simulink model "TV2016"  (Simulink 8.5)
settings: Solver=FixedStepDiscrete  StartTime=0.0  StopTime=inf  FixedStep=0.001  RelTol=1e-3
PreLoadFcn:
  | FSE_Parameters
values from neighbouring files (symbols this model uses):
  car_params = Simulink_Car_params    [TV2016_parameters.m]
  i_Diff = 15.47    [TV2016_parameters.m]
  Kp = 1    [TV2016_parameters.m]
  powerLimitControl = Simulink_el    [TV2016_parameters.m]
  settings = Simulink_Settings    [TV2016_parameters.m]
  SpdC_BCC = 0    [TV2016_parameters.m]
  Speed_Neg_sat = -21    [TV2016_parameters.m]
  Speed_Pos_sat = 21    [TV2016_parameters.m]
  speedEstimation = Simulink_speedEst    [TV2016_parameters.m]
  Tn_n = 0    [TV2016_parameters.m]
  tractionControl = Simulink_tc    [TV2016_parameters.m]
  Use_Joystick = 1    [TV2016_parameters.m]
  yawRateControl = Simulink_yawRate    [TV2016_parameters.m]
libraries: CarMaker4SL x174, simulink x27, simulink_extras x14
(part 5 of 5)

== matlab function CarMaker/Estimations/EstimateVx/velocity_Estimation ==
  data: sensors input Bus: SensorInputs; V_est_x output double; normalForces input Bus: normalForces; settings parameter double; car_params parameter double; speedEstimation parameter double
function V_est_x  = velocityEstimation(sensors,normalForces,settings,car_params,speedEstimation)
%#codegen


persistent firstIteration;
persistent v;
persistent error;
persistent K;
persistent drift;

k_FL = single(0); % Gain 
k_FR = single(0); % Gain
k_RL = single(0); % Gain
k_RR = single(0); % Gain
% Gains for trusting, not trusting wheel speed measurements
Hg = speedEstimation.High_gain;
Lg = speedEstimation.Low_gain;
% Variances
all_Var = single(0); % Variance for all measurements
front_rear_Var = single(0);
front_Var = single(0);
rear_Var = single(0);
left_Var = single(0);
right_Var = single(0);
% LIMITS:
velocity_deviation_limit = speedEstimation.velocity_deviation_limit;
lim = speedEstimation.variance_limit;
RPM_derivative_limit = speedEstimation.RPM_derivative_limit;

% Measurement vector
C = [1;1;1;1]; % Create four copies of predicted vx


c = single(2*pi/(car_params.GR*60));

t = settings.control_system_sample_time;
%Weights taken from wikipedia
%sg_Weight = single( [ 1; -8; 0; 8; -1] );
sg_Weight = single( [ -1; 8; 0; -8; 1] );
%sg_Weight = single([0.3; 0.1; -0.1 ; -0.3]);
%sg_Weight = single([1; -1; 0 ; -0]);
% ------------------------------
% COPY VARIABLES EACH TIMESTEP
% ------------------------------
S = sensors.steering_wheel_angle; % Steering angle in rad( Mean of front wheels)
ax = sensors.ax; % Should be true linear acceleration compensated for roll angle
%Fz, used to determine what wheel speeds to trust.
Fz = [normalForces.FL, normalForces.FR, normalForces.RL ,normalForces.RR];
% Determine CoG Vx from motor RPM. Simple atm. Not considering vy.
Whl_v_FL = sensors.RPM_FL*c*car_params.r_eff*cos(S) + sensors.yawRate*car_params.t_f;
Whl_v_FR = sensors.RPM_FR*c*car_params.r_eff*cos(S) - sensors.yawRate*car_params.t_f;
Whl_v_RL = sensors.RPM_RL*c*car_params.r_eff + sensors.yawRate*car_params.t_r;
Whl_v_RR = sensors.RPM_RR*c*car_params.r_eff - sensors.yawRate*car_params.t_r;
whl_speed.v_FL = Whl_v_FL;
whl_speed.v_FR = Whl_v_FR;
whl_speed.v_RL = Whl_v_RL;
whl_speed.v_RR = Whl_v_RR;


RPM = [sensors.RPM_FL, sensors.RPM_FR, sensors.RPM_RL, sensors.RPM_RR]';
% Measurement vector, compensated RPMS
Y_meas = [Whl_v_FL, Whl_v_FR, Whl_v_RL, Whl_v_RR]';
% Input Derivative of RPM
rateRPM_FL = sensors.RPM_der_FL;
rateRPM_FR = sensors.RPM_der_FR;
rateRPM_RL = sensors.RPM_der_RL;
rateRPM_RR = sensors.RPM_der_RR;

% Different sums of normal forces, used to determine what wheels to trust
left_Fz = sum(Fz([1 3]));
right_Fz = sum(Fz([2 4]));
front_Fz = sum(Fz(1:2));
rear_Fz = sum(Fz(3:4));
% ALGORITHM
if (isempty(firstIteration))
    K = single(ones(1,4));
    v = single(0);
    V_est_x = v;
    error = Y_meas- C*v;
    firstIteration = 2;
    drift = single(0);
else
    v_ins = sensors.V_x_INS + 0.05 + drift;
    mean_WhlV = max(0.001,mean(Y_meas));
    mean_front_WhlV = max(0.001,mean(Y_meas(1:2)));
    mean_rear_WhlV  = max(0.001,mean(Y_meas(3:4)));
    mean_left_WhlV  = max(0.001,mean(Y_meas([1 3])));
    mean_right_WhlV = max(0.001,mean(Y_meas([2 4])));

    all_Var = var(Y_meas,1)/mean_WhlV;
    front_rear_Var = var([mean_front_WhlV, mean_rear_WhlV],1)/mean_WhlV;
    front_Var = var(Y_meas(1:2),1)/mean_front_WhlV;
    rear_Var  = var(Y_meas(3:4),1)/mean_rear_WhlV;
    
    left_Var    = var(Y_meas([1 3]),1)/mean_left_WhlV;
    right_Var   = var(Y_meas([2 4]),1)/mean_right_WhlV;   
    
    if ( (abs(Whl_v_FL - v_ins) > velocity_deviation_limit)...
       && (abs(Whl_v_FR - v_ins) > velocity_deviation_limit)...
       && (abs(Whl_v_RL - v_ins) > velocity_deviation_limit)...
       && (abs(Whl_v_RR - v_ins) > velocity_deviation_limit) )
        
        K = [Lg, Lg, Lg, Lg];
    elseif (all_Var  < lim ) 
        % low variance for all wheels.
        % Check derivative of motor RPM
        if ( (rateRPM_FL > RPM_derivative_limit) ||...
             (rateRPM_FR > RPM_derivative_limit) ||...
             (rateRPM_RL > RPM_derivative_limit) ||...
             (rateRPM_RR > RPM_derivative_limit))
            K = [Lg, Lg, Lg, Lg];
        % Rate of change of RPM can be low but slip rate is large
        % Check against drifting INS velocity 
        else
            K = [Hg, Hg ,Hg ,Hg];
        end
    % Variance is high. What wheel(s) are causing this.. 
    % STRUCTURE:
    % 1 = FRONT AND REAR DIFFER
    % 2 = LEFT AND RIGHT DIFFER
    % 3 = FL WRONG
    % 4 = FR WRONG
    % 5 = RL WRONG
    % 6 = RR WRONG
    % 7 Combinations of 3-6 that are not handled in 1-2.
    
    %1: FRONT AND REAR DIFFER
    elseif( (right_Var > front_Var) && (right_Var > rear_Var)...
            && (left_Var > front_Var) && (left_Var > rear_Var))
        % High variance between front and rear, and low variance 
        % at front and rear.
        
        % Also need to check if front/rear wheels are slippin    
        % Front wheels over limit while rear is ok
        if (((rateRPM_FL > RPM_derivative_limit) ||...
             (rateRPM_FR > RPM_derivative_limit)) &&...
            ((rateRPM_RL < RPM_derivative_limit) ||...
             (rateRPM_RR < RPM_derivative_limit)) )
             
            K = [Lg, Lg, Hg, Hg];
        % Rear wheels over limit while front is ok
        elseif ( ((rateRPM_FL < RPM_derivative_limit) ||...
                 (rateRPM_FR < RPM_derivative_limit)) &&...
                ((rateRPM_RL > RPM_derivative_limit) ||...
                 (rateRPM_RR > RPM_derivative_limit)) )
             K = [Hg, Hg, Lg, Lg];
        % All are over limit
        elseif  ((rateRPM_FL > RPM_derivative_limit) &&...
                 (rateRPM_FR > RPM_derivative_limit) &&...
                 (rateRPM_RL > RPM_derivative_limit) &&...
                 (rateRPM_RR > RPM_derivative_limit) ) 
              K = [Lg, Lg, Lg, Lg];
              
        % The rate of change of RPM will flatten out and the high
        % slip ratio will still exist. Handle this
        
        % Check big difference in wheel speeds
        % Two cases. Driving and braking. 
        
        % Driving. Need logic to determine driving/braking
        elseif ( (RPM(1) + RPM(2)) > (RPM(3) + RPM(4)) )
            K = [Lg, Lg, Hg, Hg];
        elseif ( (RPM(1) + RPM(2)) < (RPM(3) + RPM(4)) )
            K = [Hg, Hg, Lg, Lg];
            % If frontFZ - rearFZ < 0, then FL is set to 0
            % Else it is set to a positive gain
%             k_FL = (1/abs(front_Fz-rear_Fz))*max(0,front_Fz - rear_Fz);
%             k_FR = (1/abs(front_Fz-rear_Fz))*max(0,front_Fz - rear_Fz);
% 
%             k_RL = (1/abs(rear_Fz-front_Fz))*max(0,rear_Fz-front_Fz)*0.5;
%             k_RR = (1/abs(rear_Fz-front_Fz))*max(0,rear_Fz-front_Fz)*0.5;
%            K = [k_FL, k_FR, k_RL, k_RR];
        end
    %2: LEFT AND RIGHT WHEELS DIFFER
    elseif ( ((front_Var > right_Var) && (rear_Var > right_Var)) ||...
            ( (front_Var > left_Var) && (rear_Var > left_Var)))
   
        k_FL = (1/abs(left_Fz-right_Fz))*max(0,left_Fz - right_Fz);
        k_RL = (1/abs(left_Fz-right_Fz))*max(0,left_Fz - right_Fz);
        
        k_FR = (1/abs(right_Fz-left_Fz))*max(0,right_Fz-left_Fz);
        k_RR = (1/abs(right_Fz-left_Fz))*max(0,right_Fz-left_Fz);
        
        K = [k_FL, k_FR, k_RL, k_RR];
        
    %3: FL WRONG
    elseif ( (left_Var > rear_Var) && (left_Var > right_Var)...
            && (front_Var > rear_Var) )
        k_FL = single(0);
        k_FR = single(0);
        k_RL = single(1);
        k_RR = single(1);
        K = [k_FL, k_FR, k_RL, k_RR];
    %4: FR WRONG
    elseif ( (right_Var > rear_Var) && (right_Var > left_Var)...
            && (front_Var > rear_Var))
        k_FL = single(0);
        k_FR = single(0);
        k_RL = single(1);
        k_RR = single(1);
        K = [k_FL, k_FR, k_RL, k_RR]; 
    %5: RL WRONG
    elseif ( (left_Var > front_Var) && (left_Var > right_Var)...
            && (rear_Var > front_Var))
        
        k_FL = single(1);
        k_FR = single(1);
        k_RL = single(0);
        k_RR = single(0);
        K = [k_FL, k_FR, k_RL, k_RR]; 
        
    %5: RR WRONG    
    elseif ( (right_Var > front_Var) && (right_Var > left_Var)...
            && (rear_Var > front_Var))
        k_FL = single(1);
        k_FR = single(1);
        k_RL = single(0);
        k_RR = single(0);
        K = [k_FL, k_FR, k_RL, k_RR]; 
    else
        k_FL = single(0);
        k_FR = single(0);
        k_RL = single(0);
        k_RR = single(0);
        K = [k_FL, k_FR, k_RL, k_RR]; 
    end
    
    drift = drift + 0.03*t;
   
    %v = v + t*ax;
    v = v + t*(ax + K*error);
    error = Y_meas - C*v ;
    V_est_x = 0.98*v;
end
end

== matlab function CarMaker/Control_System /Control /Throttle // Brake Mapping/MATLAB Function ==
  data: states input double; settings parameter double; T_req output double; car_params parameter double
function T_req = pedalMapping(states,settings,car_params)
%#codegen

    KERS_pos = states.KERS_pos;
    throttle = states.Input_throttle;
    T_req = single(0);
    Fx_req = single(0);
    max_drive_torque = settings.max_motor_torque*4;
    max_brake_torque = settings.max_motor_brake_torque*4;
    
   persistent firstIteration;
   persistent KERS_allowed;
   persistent torque_request_derating;
   
   % Hysteresis on KERS pedal input to avoid oscillation around 
   % allowed KERS speed. 
   if isempty(firstIteration)
      firstIteration = 2; % Avoid overflow in the register and count 1 again
      KERS_allowed = uint32(0);
   else
       
       % EVALUATE THE CASE WHEN TRACTION CONTROL IS NOT ON AND ALOT OF KERS
       % AND FRICTION BRAKING IS APPLIED -> WHEEL RPM < KERS LIMIT -> KERS
       % RELEASES, BUT FRICTION BRAKING IS NOT ENOUGH TO KEEP WHEEL
       % LOCKED-> WHEEL > KERS LIMIT -> MAXIMUM KERS IS APPLIED AGAIN ->
       % REPEAT... 
       
       % Hysteresis around the minimum KERS speed
       if     ( (KERS_allowed == 0) && (states.V_x > settings.KERS_speed_limit_hyst_high) )
           KERS_allowed = uint32(1);
       elseif ( (KERS_allowed == 1) && (states.V_x < settings.KERS_speed_limit_hyst_low) )
           KERS_allowed = uint32(0);
       end
       % Hysteresis around maximum allowable RPM.
       % The problem is if the motor RPM increases beyond a set limit,
       % around 20k RPM, as no direct speed control is done by the inverter
       % (as we bypass the speed controller). 
       
       % Find a solution that prohibits (too large) torque requests to the inverters at
       % some RPM limit without oscillating
       
       % The speed limit set in the inverters must be the last line of
       % defense (as it disabled output stage). While the solution implemented here must be the first. 
       
       % Perhaps start a torque request derating at LIMIT_START, which at
       % LIMIT_END equals just enough torque to maintain top speed.. 
       
       % Maxmotortorque calculation used in torque allocation will already
       % limit torque to maximum 10-14 Nm for each motor. 
       
       % I think we should test maximum acceleration while monitoring Max
       % RPM and evaluate if this is even a case... 
         
       
   end   
     
  if (settings.KERS_active == 1) 
      T_req = max_drive_torque*throttle  -  max_brake_torque*KERS_pos*single(KERS_allowed);
  else
      T_req = max_drive_torque*throttle;
  end
  
     
end

== matlab function CarMaker/VehicleControl/CreateBus VhclCtrl/Add KERS ==
  data: brake_pedal input double; KERS_pos output double; brake_pos output double
function [KERS_pos, brake_pos] = fcn(brake_pedal)
%#codegen

% 0-0.5 = KERS , 0.5-1.0 = 0-1 brake
    KERS_pos = single(0);
    brake_pos = 0;
    if brake_pedal >= 0 & brake_pedal <=  0.5
        KERS_pos = single(2*brake_pedal);
        brake_pos = 0;
    else
        KERS_pos = single(1);
        brake_pos = 2*(brake_pedal -0.5);
    end
    
%     if brake_pedal >= 0 & brake_pedal <=  1.0001
%         KERS_pos = single(brake_pedal);
%         brake_pos = 0;
%     else
%         KERS_pos = single(1);
%         brake_pos = 2*(brake_pedal -0.5);
%     end


end

== matlab function CarMaker/Estimations/SR_Calculation/Slip ratio ==
  data: V_x input double; SR output Bus: SR; whl_v input Bus: Whl_speed; sensor input double; car_params parameter double
function SR = slipRatioCalculation(V_x,whl_v,sensor,car_params)
%#codegen

c = single(2*pi/60);
ax = sensor.ax;

omega_der_FL = sensor.RPM_der_FL*c;
omega_FL = sensor.RPM_FL*c;

SR.FL = single((whl_v.FL - V_x) / max([0.01, abs(whl_v.FL), abs(V_x)]));
SR.FR = single((whl_v.FR - V_x) / max([0.01, abs(whl_v.FR), abs(V_x)]));
SR.RL = single((whl_v.RL - V_x) / max([0.01, abs(whl_v.RL), abs(V_x)]));
SR.RR = single((whl_v.RR - V_x) / max([0.01, abs(whl_v.RR), abs(V_x)]));

% if (abs(whl_v.FL) >= abs(V_x))
%     SR_der.FL = (-ax*omega_FL + omega_der_FL*V_x)/(car_params.r_eff*omega_FL^2);
% else
%     SR_der.FL = single(0);
% end





%SR_Kp = tractionControl.Kp;
%SR_Ki = tractionControl.Ki;

%speed = states.V_x;
% if (states.V_x < 1) 
%     SR_Kp = single(5);
%     SR_Ki = single(0);
% else
%     SR_Kp = single(5);
%     SR_Ki = single(200);
% end

end

== matlab function CarMaker/Estimations/RPM_to_linearVelocity/whl_v_calculation ==
  data: sensors input Bus: SensorInputs; meanWheelAngle input double; car_params parameter double; whl_speed output Bus: Whl_speed
function whl_speed = rpmToWhlVelocity(sensors,meanWheelAngle,car_params)
%#codegen


S = meanWheelAngle; % Steering angle in rad( Mean of front wheels)
c = single(2*pi/(car_params.GR*60));

% Determine CoG Vx from motor RPM. Simple atm. Not considering vy.
whl_speed.FL = sensors.RPM_FL*c*car_params.r_eff*cos(S) + sensors.yawRate*car_params.t_f;
whl_speed.FR = sensors.RPM_FR*c*car_params.r_eff*cos(S) - sensors.yawRate*car_params.t_f;
whl_speed.RL = sensors.RPM_RL*c*car_params.r_eff        + sensors.yawRate*car_params.t_r;
whl_speed.RR = sensors.RPM_RR*c*car_params.r_eff        - sensors.yawRate*car_params.t_r;

== matlab function CarMaker/Estimations/Fx_Estimation/EstimateFx ==
  data: car_params parameter double; Fx output Bus: Fx; sensors input Bus: SensorInputs; T_CM input Bus: T_meas
function Fx = estimateFx(car_params, sensors, T_CM)
%#codegen
Iq_FL = sensors.Iq_FL;
Iq_FR = sensors.Iq_FR;
Iq_RL = sensors.Iq_RL;
Iq_RR = sensors.Iq_RR;

Id_FL = sensors.Id_FL;
Id_FR = sensors.Id_FR;
Id_RL = sensors.Id_RL;
Id_RR = sensors.Id_RR;

Kt = car_params.Kt;     % Torque constant
Lq = car_params.Lq;     % Quadrature axis inductance 
Ld = car_params.Ld;     % Direct access inductance
Jw = car_params.Jw;     % Motor inertia
R  = car_params.r_eff;  % Radius center of rim to tire contact
GR = car_params.GR;     % Gear ratio
% Convert RPM Derivative to angular acceleration
c = single(2*pi/(GR*60));
ang_acc_FL = c*sensors.RPM_der_FL;
ang_acc_FR = c*sensors.RPM_der_FR;
ang_acc_RL = c*sensors.RPM_der_RL;
ang_acc_RR = c*sensors.RPM_der_RR;

%T_FL = (Iq_FL*Kt*sqrt(2)-(Lq-Ld)*Id_FL)*GR;
%T_FR = (Iq_FR*Kt*sqrt(2)-(Lq-Ld)*Id_FR)*GR;
%T_RL = (Iq_RL*Kt*sqrt(2)-(Lq-Ld)*Id_RL)*GR;
%T_RR = (Iq_RR*Kt*sqrt(2)-(Lq-Ld)*Id_RR)*GR;
T_FL = T_CM.FL;
T_FR = T_CM.FR;
T_RL = T_CM.RL;
T_RR = T_CM.RR;



Fx.FL = (T_FL - Jw*ang_acc_FL)/R;
Fx.FR = (T_FR - Jw*ang_acc_FR)/R;
Fx.RL = (T_RL - Jw*ang_acc_RL)/R;
Fx.RR = (T_RR - Jw*ang_acc_RR)/R;

== matlab function CarMaker/Estimations/friction_estimation/estimateFrictionCoefficient ==
  data: Fx input Bus: Fx; mu output double; Fz input Bus: normalForces; SR input Bus: SR; settings parameter double; normLongTireForce output Bus: normLongTireForce
function [mu, normLongTireForce]= estimateFrictionCoefficient(Fx,Fz,SR,settings)
%#codegen
persistent mu_FL;
persistent mu_FR;
persistent mu_RL;
persistent mu_RR;

persistent firstIteration;

if isempty(firstIteration)
    firstIteration = 2; %
    mu_FL = settings.mu;
    mu_FR = settings.mu;
    mu_RL = settings.mu;
    mu_RR = settings.mu;
    normLongTireForce.FL = single(0);
    normLongTireForce.FR = single(0);
    normLongTireForce.RL = single(0);
    normLongTireForce.RR = single(0);
else
    normLongTireForce.FL = (Fx.FL/Fz.FL);
    normLongTireForce.FR = (Fx.FR/Fz.FR);
    normLongTireForce.RL = (Fx.RL/Fz.RL);
    normLongTireForce.RR = (Fx.RR/Fz.RR);
    
    if (SR.FL > 0.09) && (SR.FL < 0.13)
        mu_FL = max( (Fx.FL/Fz.FL), mu_FL);
    end
    if (SR.FR > 0.09) && (SR.FR < 0.15)
        mu_FR = max( (Fx.FR/Fz.FR), mu_FR);
    end

    if (SR.RL > 0.09) && (SR.RL < 0.15)
        mu_RL = max( (Fx.RL/Fz.RL), mu_RL);
    end

    if (SR.RR > 0.09) && (SR.RR < 0.15)
       mu_RR = max( (Fx.RR/Fz.RR), mu_RR);
    end
end


mu = (mu_FL + mu_FR + mu_RL + mu_RR) / 4;

end

== matlab function CarMaker/VehicleControl/CreateBus VhclCtrl/RacingwheelInterface/Add KERS ==
  data: brake_pedal input double; KERS_pos output double; brake_pos output double
function [KERS_pos, brake_pos] = fcn(brake_pedal)
%#codegen

% 0-0.5 = KERS , 0.5-1.0 = 0-1 brake
    KERS_pos = single(0);
    brake_pos = 0;
    if (brake_pedal > 0) && (brake_pedal <  0.5)
        KERS_pos = single(2*brake_pedal);
        brake_pos = 0;
    else
        KERS_pos = single(1);
        brake_pos = 2*(brake_pedal -0.5);
    end
    
%     if brake_pedal >= 0 & brake_pedal <=  1.0001
%         KERS_pos = single(brake_pedal);
%         brake_pos = 0;
%     else
%         KERS_pos = single(1);
%         brake_pos = 2*(brake_pedal -0.5);
%     end


end

== matlab function CarMaker/Control_System /Control /Slip Rate Control /Traction Controllers/MATLAB Function ==
  data: Ti_FL input double; Ti_FR input double; Ti_lim output Bus: Ti_lim; Ti_RL input double; Ti_RR input double; TC_FL input double; TC_FR input double; TC_RL input double; TC_RR input double; states input Bus: States; T_req input double
function Ti_lim =  TCOutputHandling(Ti_FL, Ti_FR, Ti_RL, Ti_RR, TC_FL,TC_FR,TC_RL,TC_RR,states, T_req)
%#codegen

yawRate_p_lim = 0.3;
ay_p_lim = 3;

straightline = uint32(0);

if ( (states.r > -yawRate_p_lim) && (states.r < yawRate_p_lim) &&...
     (states.ay > -ay_p_lim) && (states.ay < ay_p_lim) )
    straightline = 1;
else
    straightline = 0;
end


% FRONT SIDE
n_cmp = single(-0.03);
p_cmp = single(0.03);

% If driving ~ straightline then couple the outputs
% Else, each TC works individually. 
if      ( (straightline == 1) && (T_req > p_cmp) )
    % Couple TC outputs to maintain stability on mu split surfaces 
    % under acceleration and deceleration
    Ti_lim.FL = max(0, (Ti_FL + min(TC_FL,TC_FR)));
    Ti_lim.FR = max(0, (Ti_FR + min(TC_FL,TC_FR)));  
    
    Ti_lim.RL = max(0, (Ti_RL + min(TC_RL,TC_RR)));
    Ti_lim.RR = max(0, (Ti_RR + min(TC_RL,TC_RR)));
 
elseif  ( (straightline == 1) && (T_req < n_cmp) )
    % Couple TC outputs to maintain stability on mu split surfaces 
    % under acceleration and deceleration
    Ti_lim.FL = min(0, (Ti_FL + max(TC_FL,TC_FR) ) );   
    Ti_lim.FR = min(0, (Ti_FR + max(TC_FL,TC_FR) ) );    
    Ti_lim.RL = min(0, (Ti_RL + max(TC_RL,TC_RR) ) );
    Ti_lim.RR = min(0, (Ti_RR + max(TC_RL,TC_RR) ) );   
else
    % Decouple TC outputs to avoid interferring too much with the stability
    % of the vehicle while cornering. This is the DYC systems job. 
    Ti_lim.FL = Ti_FL + TC_FL;
    Ti_lim.FR = Ti_FR + TC_FR;
    Ti_lim.RL = Ti_RL + TC_RL;
    Ti_lim.RR = Ti_RR + TC_RR;
end

end

== matlab function CarMaker/Control_System /Control /Slip Rate Control /SMC Traction Control/MATLAB Function ==
  data: Ti_FL input double; Ti_FR input double; Ti_lim output Bus: Ti_lim; Ti_RL input double; Ti_RR input double; TC_FL input double; TC_FR input double; TC_RL input double; TC_RR input double; states input Bus: States; T_req input double
function Ti_lim =  TCOutputHandling(Ti_FL, Ti_FR, Ti_RL, Ti_RR, TC_FL,TC_FR,TC_RL,TC_RR,states, T_req)
%#codegen

yawRate_p_lim = 0.2;
ay_p_lim = 3;

straightline = uint32(0);

if ( (states.r > -yawRate_p_lim) && (states.r < yawRate_p_lim) && ...
     (states.ay > -ay_p_lim) && (states.ay < ay_p_lim) )
    straightline = 1;
else
    straightline = 0;
end


% Proposal : TC only active if yaw rate within some set

% FRONT SIDE
n_cmp = single(-0.03);
p_cmp = single(0.03);

% If driving ~ straightline then couple the outputs
% Else, each TC works individually. 
if      ( (straightline == 1) && (T_req > p_cmp) )
    % Couple TC outputs to maintain stability on mu split surfaces 
    % under acceleration and deceleration
    Ti_lim.FL = max(0, (Ti_FL + min(TC_FL,TC_FR) ) );
    Ti_lim.FR = max(0, (Ti_FR + min(TC_FL,TC_FR) ) );
    
    Ti_lim.RL = max(0, (Ti_RL + min(TC_RL,TC_RR) ) );
    Ti_lim.RR = max(0, (Ti_RR + min(TC_RL,TC_RR) ) );
 
elseif  ( (straightline) && (T_req < n_cmp) )
    % Couple TC outputs to maintain stability on mu split surfaces 
    % under acceleration and deceleration
    Ti_lim.FL = min(0, (Ti_FL + max(TC_FL,TC_FR) ) );
    Ti_lim.FR = min(0, (Ti_FR + max(TC_FL,TC_FR) ) );
    
    Ti_lim.RL = min(0, (Ti_RL + max(TC_RL,TC_RR) ) );
    Ti_lim.RR = min(0, (Ti_RR + max(TC_RL,TC_RR) ) );   
else
    % Decouple TC outputs to avoid interferring too much with the stability
    % of the vehicle while cornering. This is the DYC systems job. 
    Ti_lim.FL = Ti_FL + TC_FL;
    Ti_lim.FR = Ti_FR + TC_FR;
    Ti_lim.RL = Ti_RL + TC_RL;
    Ti_lim.RR = Ti_RR + TC_RR;
end

end




% if      ( (TC_FL < n_cmp) && (TC_FR < n_cmp) )
%     % add the most negative
% elseif  ( (TC_FL > p_cmp) && (TC_FR > p_cmp) )
%     % Add the most positive
%     
% elseif  ( (TC_FL < n_cmp) && (TC_FR > p_cmp) )
%     % Individual control
% elseif  ( (TC_FL > p_cmp) && (TC_FR < n_cmp) )
%     % Individual control
%     
%     
% elseif  ( (TC_FL > p_cmp) && (TC_FR < p_cmp) && (TC_FR > n_cmp) && (T_req < n_cmp) )
%     % One wants to add, other is fine and T_req < 0 which means it must be
%     % braking either straight or into a corner.. Add to both wheels, but do
%     % not exceed 0 torque.
%     
% elseif  ( (TC_FL < p_cmp) && (TC_FL > n_cmp) && (TC_FR > p_cmp)  && (T_req < n_cmp) )
%     % One wants to add, other is fine and T_req < 0 which means it must be
%     % braking either straight or into a corner.. Add to both wheels, but do
%     % not exceed 0 torque.    
%     
% elseif  ( (TC_FL < n_cmp) && ( (TC_FR < p_cmp) && (TC_FR > n_cmp) ) ...
%           && (T_req > p_cmp) && (straightline))
%     % One wants to subtract, other is fine and T_req > 0 and straightline
%     % which means mu split acceleration.
%     
%  elseif  ( (TC_FL > n_cmp) && (TC_FL < p_cmp) && (TC_FR < n_cmp) ) ...
%           && (T_req > p_cmp) && (straightline))
%     % One wants to subtract, other is fine and T_req > 0 and straightline
%     % which means mu split acceleration.    
%     
% elseif  ( (TC_FL < n_cmp) &&  (TC_FR < p_cmp) && (TC_FR > n_cmp) ...
%            && (not(straightline)))
%     % One wants to subtract, other is fine and T_req > 0 and straightline
%     % is false which means
%     
%  elseif  ( (TC_FL > n_cmp) && (TC_FL < p_cmp) && (TC_FR < n_cmp)  ...
%            && (not(straightline)))
%     % One wants to subtract, other is fine and T_req > 0 and straightline
%     % which means mu split acceleration.       
% elseif  
%     
%     
% y = u;

== matlab function CarMaker/Control_System /Control /Slip Rate Control /SMC Traction Control/MATLAB Function1 ==
  data: states input Bus: States; SR_FL output double; SR_FR output double; SR_RL output double; SR_RR output double; vx output double
function [SR_FL,SR_FR,SR_RL,SR_RR,vx] = extractSlipRatios(states)
%#codegen


SR_FL = states.SR_FL;
SR_FR = states.SR_FR;
SR_RL = states.SR_RL;
SR_RR = states.SR_RR;

vx = states.V_x;

== matlab function CarMaker/RPM_Derivative/Compute Derivative of RPM ==
  data: sensors input double; RPMDerivative output Bus: RPMDerivative; settings parameter double
function RPMDerivative ...
          = computeRPMDerivative(sensors,settings)
%#codegen
RPM_FL = sensors.RPM_FL;
RPM_FR = sensors.RPM_FR;
RPM_RL = sensors.RPM_RL;
RPM_RR = sensors.RPM_RR;



t = settings.control_system_sample_time;
sg_Weight = single( [ -1; 8; 0; -8; 1] );

nr_Coefficients = uint32(5);
persistent firstIteration;
persistent frame;
persistent RPM_prev_FL;
persistent RPM_prev_FR;
persistent RPM_prev_RL;
persistent RPM_prev_RR;

RPMDerivative.FL = single(0);
RPMDerivative.FR = single(0);
RPMDerivative.RL = single(0);
RPMDerivative.RR = single(0);


if isempty(firstIteration)
        firstIteration = 2;
        RPM_prev_FL = RPM_FL;
        RPM_prev_FR = RPM_FR;
        RPM_prev_RL = RPM_RL;
        RPM_prev_RR = RPM_RR;
        
        frame = single(zeros(1,nr_Coefficients));
        RPMDerivative.FL = single(0);
        RPMDerivative.FR = single(0);
        RPMDerivative.RL = single(0);
        RPMDerivative.RR = single(0);

else
    RPMDerivative.FL = abs( (RPM_FL - RPM_prev_FL)/(t));
    RPMDerivative.FR = abs( (RPM_FR - RPM_prev_FR)/(t));
    RPMDerivative.RL = abs( (RPM_RL - RPM_prev_RL)/(t));
    RPMDerivative.RR = abs( (RPM_RR - RPM_prev_RR)/(t));
    
    RPM_prev_FL = RPM_FL;
    RPM_prev_FR = RPM_FR;
    RPM_prev_RL = RPM_RL;
    RPM_prev_RR = RPM_RR;
end

end

    
    
%     frame = [RPM, frame(1:(end-1))]    
%     %Calculate output
%     rateRPM = abs((frame*weight_Vector)./(12*ts));

== matlab function CarMaker/Control_System /Control /Slip Rate Control /SMC Traction Control/Slip Rate FL/SMC ==
  data: muOfSlip input double; TC output double; SR input double; SR_ref input double; car_params parameter double; states input double; K input double
function TC = fcn(muOfSlip,SR,SR_ref,car_params, states,K)
%#codegen
Jr = 0.2;
GR = car_params.GR;
r = car_params.r_eff;
m = car_params.mass;
Fz_FL = states.Fz_FL;
%slip = ((Jr/(m*r^2*(1-SR))) +1 )*muOfSlip*Fz_FL*r

ySlip = (r*(1-SR)^2)/(Jr*states.V_x);
force = muOfSlip*Fz_FL*r/GR
TC = force - (K/(ySlip))*sign(SR-SR_ref)*min(1,abs(SR-SR_ref));

== matlab function CarMaker/Control_System /Control /Slip Rate Control /SMC Traction Control/Slip Rate FL1/SMC ==
  data: muOfSlip input double; TC output double; SR input double; SR_ref input double; car_params parameter double; states input double; K input double
function TC = fcn(muOfSlip,SR,SR_ref,car_params, states,K)
%#codegen
Jr = 0.2;
GR = car_params.GR;
r = car_params.r_eff;
m = car_params.mass;
Fz_FR = states.Fz_FR;
%slip = ((Jr/(m*r^2*(1-SR))) +1 )*muOfSlip*Fz_FL*r
ySlip = (r*(1-SR)^2)/(Jr*states.V_x);
force = muOfSlip*Fz_FR*r/GR
TC = force - (K/(ySlip))*sign(SR-SR_ref)*min(1,abs(SR-SR_ref));

== matlab function CarMaker/Control_System /Control /Slip Rate Control /SMC Traction Control/Slip Rate FL2/SMC ==
  data: muOfSlip input double; TC output double; SR input double; SR_ref input double; car_params parameter double; states input double; K input double
function TC = fcn(muOfSlip,SR,SR_ref,car_params, states,K)
%#codegen
Jr = 0.2;
GR = car_params.GR;
r = car_params.r_eff;
m = car_params.mass;
Fz_RL = states.Fz_RL;
%slip = ((Jr/(m*r^2*(1-SR))) +1 )*muOfSlip*Fz_FL*r
ySlip = (r*(1-SR)^2)/(Jr*states.V_x);
force = muOfSlip*Fz_RL*r/GR
TC = force - (K/(ySlip))*sign(SR-SR_ref)*min(1,abs(SR-SR_ref));

== matlab function CarMaker/Control_System /Control /Slip Rate Control /SMC Traction Control/Slip Rate FL3/SMC ==
  data: muOfSlip input double; TC output double; SR input double; SR_ref input double; car_params parameter double; states input double; K input double
function TC = fcn(muOfSlip,SR,SR_ref,car_params, states,K)
%#codegen
Jr = 0.2;
GR = car_params.GR;
r = car_params.r_eff;
m = car_params.mass;
Fz_RR = states.Fz_RR;
%slip = ((Jr/(m*r^2*(1-SR))) +1 )*muOfSlip*Fz_FL*r
ySlip = (r*(1-SR)^2)/(Jr*states.V_x);
force = muOfSlip*Fz_RR*r/GR
TC = force - (K/(ySlip))*sign(SR-SR_ref)*min(1,abs(SR-SR_ref));

== matlab function CarMaker/Estimations/calculateMeanWheelAngle/calculateWheelangleandSpeed ==
  data: mean_wheel_angle output single; sensor input Bus: SensorInputs; mean_wheel_speed output single
function [mean_wheel_angle, mean_wheel_speed] = calculateWheelAngle(sensor)
%#codegen

% Right now assumes rad for angle, and rad/s for speed
mean_wheel_angle    = single(0.2536*sensor.steering_wheel_angle);
mean_wheel_speed    = single(0.2536*sensor.steering_wheel_speed);

end

== matlab function CarMaker/Estimations/Fz_Estimation/FzEstDamper ==
  data: sensors input Bus: SensorInputs; Fz_damp_FL input double; Fz_damp_FR input double; Fz_damper_est output Bus: normalForces; Fz_damp_RL input double; Fz_damp_RR input double; car_params parameter double
function Fz_damper_est =  FzEstDamp(sensors, Fz_damp_FL, Fz_damp_FR, Fz_damp_RL, Fz_damp_RR, car_params)
%#codegen

Ks_front    = car_params.spring_constant_front;
Ks_rear     = car_params.spring_constant_rear;

MR_front    = car_params.motion_ratio_front;
MR_rear     = car_params.motion_ratio_rear;     


Fz_damper_est.FL = (Ks_front*sensors.damper_pos_FL + Fz_damp_FL)*MR_front;
Fz_damper_est.FR = (Ks_front*sensors.damper_pos_FR + Fz_damp_FR)*MR_front;
Fz_damper_est.RL = (Ks_rear*sensors.damper_pos_RL + Fz_damp_RL)*MR_rear;
Fz_damper_est.RR = (Ks_rear*sensors.damper_pos_RR + Fz_damp_RR)*MR_rear;

== matlab function CarMaker/Control_System /Control /Torque allocation /Torque Allocation/TorqueAllocation ==
  data: Ti_lim output Bus: Ti_lim; T_req input double; states input double; maxMotorTorque input double; settings parameter double; car_params parameter double; Mz_ref input double; Ti_max output double; Mz_error output double; Mz_allocated output double; yawRateControl parameter double
function [Ti_lim,Ti_max,Mz_error, Mz_allocated]  = torqueAllocation(T_req,states,maxMotorTorque,settings, car_params, Mz_ref,yawRateControl)
%#codegen
%STATES
r = states.r;
negative_torque_limit = yawRateControl.negative_torque_limit;

%PARAMETERS
%mu = states.mu;
mu = settings.mu;
tf = car_params.t_f*2;
tr = car_params.t_r*2;
GR = car_params.GR;
r_eff = car_params.r_eff;
R = [r_eff; r_eff; r_eff; r_eff]';
%Load Transfer
Fzi = [max(1,states.Fz_FL) max(1,states.Fz_FR) max(1,states.Fz_RL) max(1,states.Fz_RR)]';
alfa_r =  (Fzi(3) + Fzi(4)) / (Fzi(1) + Fzi(2) + Fzi(3) + Fzi(4));
%MZ
S = states.wheel_angle;

l1 = car_params.t_f*cos(S);
l2 = car_params.t_f*cos(S);
l3 = car_params.t_r;
l4 = car_params.t_r;
L = [-l1; l2; -l3; l4];



%FIND MAXIMUM ALLOWED MOTOR TORQUE, TIRE/MOTOR
Ti_max          = single(zeros(4,1));
Ti_max_tire     = single(zeros(4,1));

RPM = [states.RPM_FL, states.RPM_FR, states.RPM_RL, states.RPM_RR];
Ti_max_motor = [maxMotorTorque.mmt_FL,maxMotorTorque.mmt_FR,maxMotorTorque.mmt_RL,maxMotorTorque.mmt_RR]; 

%Tire saturation based on mu and Fz
for i=1:4
    Ti_max_tire(i) = Fzi(i)*mu*R(i)/GR;
end


% Find minimum of tire saturation Torque and motor
for i=1:4
    Ti_max(i) = min(Ti_max_tire(i), Ti_max_motor(i));
end
%**********************************************%

T_F = single(zeros(2,1));
T_R = single(zeros(2,1));
sat_F = uint32(0);
sat_R = uint32(0);

if ( T_req >= 0)
    switch settings.TV_Method
        case 1
            % Only positive Torque
            [T_F, sat_F] = allocatePositiveTorque(Ti_max(1), Ti_max(2), T_req, R(1), R(2), (1-alfa_r), Mz_ref, GR, tf);
            [T_R, sat_R] = allocatePositiveTorque(Ti_max(3), Ti_max(4), T_req, R(3), R(4), alfa_r, Mz_ref, GR, tr);
        case 2
            % Can also allocate negative torque
            [T_F, sat_F] = allocateTorque(Ti_max(1), Ti_max(2), T_req, R(1), R(2), (1-alfa_r), Mz_ref, GR, tf, negative_torque_limit);
            [T_R, sat_R] = allocateTorque(Ti_max(3), Ti_max(4), T_req, R(3), R(4), alfa_r, Mz_ref, GR, tr ,negative_torque_limit);
        case 3
            % Static 25 percent to each wheel
            T_F = [0.25*T_req; 0.25*T_req];
            T_R = [0.25*T_req; 0.25*T_req];
        case 4
            % Allocation with negative torque, but does not use Fz
            [T_F, sat_F] = allocateTorque(Ti_max_motor(1), Ti_max_motor(2), T_req, R(1), R(2), (1-alfa_r), Mz_ref, GR, tf, negative_torque_limit);
            [T_R, sat_R] = allocateTorque(Ti_max_motor(3), Ti_max_motor(4), T_req, R(3), R(4), alfa_r, Mz_ref, GR, tr ,negative_torque_limit);
    end
            
    if ( (sat_F == 1) && (sat_R == 1) )
        % Nothing more to do
    elseif ( (sat_F == 1) && (sat_R == 0) )     
         if ( T_F(1) < 0) 
            T_remaining = T_req - (T_F(2));
         elseif (T_F(2) < 0) 
             T_remaining = T_req - (T_F(1));
         else
             T_remaining = T_req - (T_F(1) + T_F(2));
         end
         
         if (yawRateControl.enable == 1)
             Mz_remaining = Mz_ref - (-l1*GR*T_F(1)/R(1) + l2*GR*T_F(2)/R(2));
         else
             Mz_remaining = single(0);
         end 
         
        switch settings.TV_Method
            case 1
                % Only positive Torque
                [T_R sat_R] = allocatePositiveTorque(Ti_max(3), Ti_max(4), T_remaining, R(3), R(4), 1 , Mz_remaining, GR, tr);
            case 2
                % Can also allocate negative torque
                [T_R sat_R] = allocateTorque(Ti_max(3), Ti_max(4), T_remaining, R(3), R(4), 1 , Mz_remaining, GR, tr,negative_torque_limit);
            case 4
                [T_R sat_R] = allocateTorque(Ti_max_motor(3), Ti_max_motor(4), T_remaining, R(3), R(4), 1 , Mz_remaining, GR, tr,negative_torque_limit);
        end 
    elseif ( (sat_F == 0) && (sat_R == 1) )
         if ( T_R(1) < 0) 
            T_remaining = T_req - (T_R(2));
         elseif (T_R(2) < 0) 
             T_remaining = T_req - (T_R(1));
         else
             T_remaining = T_req - (T_R(1) + T_R(2));
         end        
        % For example rear is saturated, and front can still use more torque
        %T_remaining = T_req - (T_R(1) + T_R(2));
        if (yawRateControl.enable == 1)
             Mz_remaining = Mz_ref - (-l3*GR*T_R(1)/R(3) + l4*GR*T_R(2)/R(4));
        else
             Mz_remaining = single(0);
        end 
        %Mz_remaining = Mz_ref*(1-alfa_r);
        switch settings.TV_Method
            case 1
                % Only positive Torque
                 [T_F sat_F] = allocatePositiveTorque(Ti_max(1), Ti_max(2), T_remaining, R(1), R(2), 1 , Mz_remaining, GR, tf);
            case 2
                % Can also allocate negative torque
                [T_F sat_F] = allocateTorque(Ti_max(1), Ti_max(2), T_remaining, R(1), R(2), 1 , Mz_remaining, GR, tf,negative_torque_limit);
            case 4
                [T_F sat_F] = allocateTorque(Ti_max_motor(1), Ti_max_motor(2), T_remaining, R(1), R(2), 1 , Mz_remaining, GR, tf,negative_torque_limit);
        end      
    else
        %both false
        % Nothing to do here either
    end
else
    %REGENERATIVE BRAKE COMMAND ( T_DRIVER_REQ < 0 )
    switch settings.TV_Method
        case 1
            % Only positive Torque
            [T_F, sat_F] = allocateKersTorque(Ti_max(1), Ti_max(2), T_req, R(1), R(2), (1-alfa_r), Mz_ref, GR, tf);
            [T_R, sat_R] = allocateKersTorque(Ti_max(3), Ti_max(4), T_req, R(3), R(4), alfa_r, Mz_ref, GR, tr);
            
        case 2
            % Can also allocate negative torque
            [T_F, sat_F] = allocateKersTorque(Ti_max(1), Ti_max(2), T_req, R(1), R(2), (1-alfa_r), Mz_ref, GR, tf);
            [T_R, sat_R] = allocateKersTorque(Ti_max(3), Ti_max(4), T_req, R(3), R(4), alfa_r, Mz_ref, GR, tr);
        case 3
            % Static 25 percent to each wheel
            T_F = [0.25*T_req; 0.25*T_req];
            T_R = [0.25*T_req; 0.25*T_req];
        case 4
            % Allocation with negative torque, but does not use Fz
            [T_F, sat_F] = allocateKersTorque(Ti_max_motor(1), Ti_max_motor(2), T_req, R(1), R(2), (1-alfa_r), Mz_ref, GR, tf);
            [T_R, sat_R] = allocateKersTorque(Ti_max_motor(3), Ti_max_motor(4), T_req, R(3), R(4), alfa_r, Mz_ref, GR, tr);
    end
    if (sat_F == 1 && sat_R == 1)
        %Nothing more to do
        
    elseif (sat_F == 1 && sat_R == 0)
         T_remaining = T_req - (T_F(1) + T_F(2));
         %Disable Mz_remaining if yaw control disabled?
        if (yawRateControl.enable == 1)
             Mz_remaining = Mz_ref - (-l1*GR*T_F(1)/R(1) + l2*GR*T_F(2)/R(2));
        else
             Mz_remaining = single(0);
        end
        switch settings.TV_Method
            case 1
                % Only positive Torque
                [T_R sat_R] = allocateKersTorque(Ti_max(3), Ti_max(4), T_remaining, R(3), R(4), 1 , Mz_remaining, GR, tr);

            case 2
                % Can also allocate negative torque
                [T_R sat_R] = allocateKersTorque(Ti_max(3), Ti_max(4), T_remaining, R(3), R(4), 1 , Mz_remaining, GR, tr);
            case 3
                % Static 25 %
            case 4
                % Allocation with negative torque, but does not use Fz
                [T_R sat_R] = allocateKersTorque(Ti_max_motor(3), Ti_max_motor(4), T_remaining, R(3), R(4), 1 , Mz_remaining, GR, tr);
        end
        
    elseif (sat_F == 0 && sat_R == 1)
        %For example rear is saturated, and front can still use more torque
        T_remaining = T_req - (T_R(1) + T_R(2));
        %Mz_remaining = Mz_ref*(1-alfa_r);
        
        if (yawRateControl.enable == 1)
             Mz_remaining = Mz_ref - (-l3*GR*T_R(1)/R(3) + l4*GR*T_R(2)/R(4));
        else
             Mz_remaining = single(0);
        end
        switch settings.TV_Method
            case 1
                % Only positive Torque
                [T_F sat_F] = allocateKersTorque(Ti_max(1), Ti_max(2), T_remaining, R(1), R(2), 1 , Mz_remaining, GR, tf); 

            case 2
                % Can also allocate negative torque
                [T_F sat_F] = allocateKersTorque(Ti_max(1), Ti_max(2), T_remaining, R(1), R(2), 1 , Mz_remaining, GR, tf); 
            case 3
                % Static 25 %
            case 4
                % Allocation with negative torque, but does not use Fz
                [T_F sat_F] = allocateKersTorque(Ti_max_motor(1), Ti_max_motor(2), T_remaining, R(1), R(2), 1 , Mz_remaining, GR, tf);             
        end
    else
        %both false
        %Nothing to do here either
    end
end

Ti_all = [T_F' T_R'];

Ti_lim_struct = struct;
Ti_lim_struct.FL = Ti_all(1);
Ti_lim_struct.FR = Ti_all(2);
Ti_lim_struct.RL = Ti_all(3);
Ti_lim_struct.RR = Ti_all(4);

Ti_lim = Ti_lim_struct;

% Calculate what yaw moment that was achieved with the current 
% allocation
Fx_all = prod([Ti_all; 1./R;])*GR;
Mz_allocated = L'*Fx_all';
Mz_error = Mz_ref - Mz_allocated;
end


function [T, sat] = allocateTorque(L_max, R_max, T_req,...
          R_eff_L, R_eff_R, alfa, Mz_ref, GR, t, negative_torque_limit)
      
    T = single(zeros(2,1));
    sat = uint32(0);
    % Desired torque vectoring torque
    TV_des = abs(alfa*Mz_ref*R_eff_L/(GR*t)) + abs(alfa*Mz_ref*R_eff_R/(GR*t));
    % Take absolute value since T_req can be negative in case of KERS
    T_driver = alfa*T_req;

    if ( Mz_ref <= 0)
        % Implies that left side should realize the TV torque,
        % since only torque >= 0 is used here.
        % Mz is defined positive counter clockwise
        L = min( [TV_des, T_driver, L_max]); 
        if ( (L < TV_des) ) %&& (T_driver > 0))
            % Not fulfilled desired yaw moment
            R = - min( [(TV_des - L), R_max, negative_torque_limit]);
            T = [L;R];
        else
            max_t_add = min([(L_max-TV_des), R_max, (T_driver-L)/2]);
            L = L + max_t_add;
            R = max_t_add;
            T = [L;R];
        end
        % Floats comparison
        if ( (L + 0.001) < (T_driver))
            sat = uint32(1);
        end
        return;
    else
        R = min( [TV_des, T_driver, R_max]);
        %Max torque that can be added to both  
        if ( (R < TV_des) ) % && (T_driver > 0) )
            L = -min( [(TV_des - R), L_max,negative_torque_limit]);
            T = [L;R];
        else
            max_t_add = min([(R_max - TV_des),L_max, (T_driver-R)/2]);
            R = R + max_t_add;
            L = max_t_add;
            T = [L;R];
        end
        
        if ( (R + 0.001) < (T_driver))
            sat = uint32(1);
        end
        return;
    end
end

function [T, sat] = allocateKersTorque(L_max, R_max, T_req, R_eff_L, R_eff_R, alfa, Mz_ref, GR, t )
    T = single(zeros(2,1));
    sat = uint32(0);
    % Desired torque vectoring torque
    TV_des = abs(alfa*Mz_ref*R_eff_L/(GR*t)) + abs(alfa*Mz_ref*R_eff_R/(GR*t));
    % Take absolute value since T_req can be negative in case of KERS
    T_driver = abs(alfa*T_req);
   
    if (Mz_ref + 0.0001 >= 0)
        % Positive Mz_ref requires left side (inner wheels)
        % to brake more than the outer wheels.
        L = min( [TV_des, T_driver, L_max]);
        %Max torque that can be added to both
        if L_max < abs(TV_des)
            max_t_add = single(0);
        else
            max_t_add = min([(L_max-TV_des), R_max, (T_driver-L)/2]);
        end 
        L = - (L + max_t_add);
        R = - max_t_add;
        T = [L;R];
        % Floats comparison
        if ( (abs(L) + abs(R) + 0.001) < T_driver)
            sat = uint32(1);
        end
        return;
    else
        R = min( [abs(TV_des), T_driver, R_max]);
        %Max torque that can be added to both
        if R_max < abs(TV_des)
            max_t_add = single(0);
        else
            max_t_add = min([(R_max-abs(TV_des)), L_max, (T_driver-R)/2]);
        end
        R = - (R + max_t_add);
        L = - max_t_add;
        T = [L;R];
        % Floats comparison
        if ( (abs(L) + abs(R) + 0.001) < T_driver)
            sat = uint32(1);
        end
        return;
    end
end
function [T, sat] = allocatePositiveTorque(L_max, R_max, T_req,...
          R_eff_L, R_eff_R, alfa, Mz_ref, GR, t )
      
    T = single(zeros(2,1));
    sat = uint32(0);
    % Desired torque vectoring torque
    TV_des = abs(alfa*Mz_ref*R_eff_L/(GR*t)) + abs(alfa*Mz_ref*R_eff_R/(GR*t));
    % Take absolute value since T_req can be negative in case of KERS
    T_driver = alfa*T_req;

    if ( Mz_ref <= 0)
        % Implies that left side should realize the TV torque,
        % since only torque >= 0 is used here.
        % Mz is defined positive counter clockwise
        L = min( [TV_des, T_driver, L_max]);
        %Max torque that can be added to both
        %Skal det ikke være L < TV_des
        if L_max < abs(TV_des)
            max_t_add = single(0);
        else
            max_t_add = min([(L_max-TV_des), R_max, (T_driver-L)/2]);
        end 
        L = L + max_t_add;
        R = max_t_add;
        T = [L;R];  
        % Floats comparison
        if ( (L + R + 0.001) < (T_driver))
            sat = uint32(1);
        end
        return;
    else
        R = min( [abs(TV_des), T_driver, R_max]);
        %Max torque that can be added to both
        if R_max < abs(TV_des)
            max_t_add = single(0);
        else
            max_t_add = min([(R_max-abs(TV_des)),L_max, (T_driver-R)/2]);
        end
        R = R + max_t_add;
        L = max_t_add;
        T = [L;R];
        % Floats comparison
        if ( (L + R + 0.001) < (T_driver))
            sat = uint32(1);
        end
        return;
    end
end
